simulink model "t_type_inverter"  (R2024b)
settings: Solver=FixedStepAuto  StartTime=0.0  StopTime=0.1  RelTol=1e-3
libraries: spsIGBTDiodeLib x12, spsVoltageMeasurementLib x3, spsDCVoltageSourceLib x2, spsGroundLib x1, spsThreePhaseSeriesRLCBranchLib x1, spsThreePhaseVIMeasurementLib x1, sps_lib x1
settings Model: Creator=Eng.Abd-Elrhman Saad  LastModifiedBy=Eng.Abd-Elrhman Saad

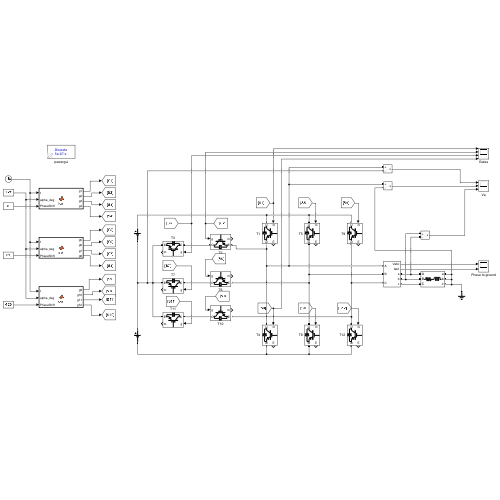
[thumbnail: Simulink's stored preview of the top-level diagram]
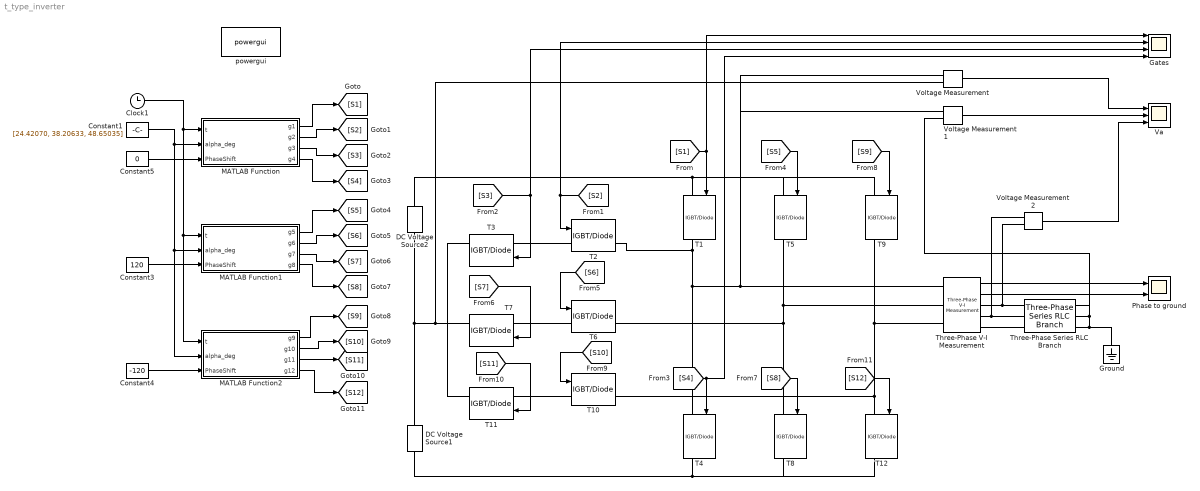
== system t_type_inverter ==
  Clock1 : Clock
  Constant1 : Constant  Value=[24.42070, 38.20633, 48.65035]
  Constant3 : Constant  Value=120
  Constant4 : Constant  Value=-120
  Constant5 : Constant  Value=0
  DC Voltage Source1 : spsDCVoltageSourceLib/DC Voltage Source  Amplitude=400  Measurements=None
  DC Voltage Source2 : spsDCVoltageSourceLib/DC Voltage Source  Amplitude=400  Measurements=None
  Gates : Scope  NumInputPorts=4
  Ground : spsGroundLib/Ground  LConnTagsString=a
  MATLAB Function : MATLAB Function  TreatAsAtomicUnit=on
  MATLAB Function1 : MATLAB Function  TreatAsAtomicUnit=on
  MATLAB Function2 : MATLAB Function  TreatAsAtomicUnit=on
  Phase to ground : Scope  NumInputPorts=2
  T{1..12} (12 alike) : spsIGBTDiodeLib/IGBT//Diode  Ron=1e-3  Rs=1e5  Cs=inf  Measurements=on
  Three-Phase Series RLC Branch : spsThreePhaseSeriesRLCBranchLib/Three-Phase Series RLC Branch  LConnTagsString=A|B|C  RConnTagsString=A|B|C  BranchType=RL  Resistance=7.07  Inductance=0.0225  Capacitance=1e-6  Measurements=None
  Three-Phase V-I Measurement : spsThreePhaseVIMeasurementLib/Three-Phase V-I Measurement  VoltageMeasurement=phase-to-ground  SetLabelV=off  LabelV=Vabc  Vpu=off  VpuLL=off  CurrentMeasurement=yes  SetLabelI=off  LabelI=Iabc  Ipu=off  Pbase=100e6  Vbase=500e3  OutputType=Complex  PhasorSimulation=off  PSBequivalent=0
  Va : Scope  NumInputPorts=3
  Voltage Measurement : spsVoltageMeasurementLib/Voltage Measurement  PhasorSimulation=off  OutputType=Complex  PSBequivalent=0
  Voltage Measurement1 : spsVoltageMeasurementLib/Voltage Measurement  PhasorSimulation=off  OutputType=Complex  PSBequivalent=0
  Voltage Measurement2 : spsVoltageMeasurementLib/Voltage Measurement  PhasorSimulation=off  OutputType=Complex  PSBequivalent=0
  powergui : sps_lib/powergui  Priority=1  SimulationMode=Discrete  SampleTime=5e-7  frequency=60  Iterations=50  frequencyindice=0  Pbase=100e6  ErrMax=1e-4  UnitsV=kV  UnitsW=MW  buscounter=0  FunctionMessages=off  echomessages=off  EnableUseOfTLC=off  CurrentSourceSwitches=off  DisableSnubberDevices=off  DisableRonSwitches=off  DisableVfSwitches=off  DisplayEquations=off  AutomaticDiscreteSolvers=off  SolverType=Tustin/Backward Euler (TBE)  Interpol=off  ExternalGateDelay=off  methode=off  Ts=100  x0status=blocks  SPID=on  SwTol=0  HookPort=off  NonlinearTolerance=1e-4  nMaxIteration=100  ContinueOnMaxIteration=off  RestoreLinks=warning  ResistiveCurrentMeasurement=off  Frange=[0:2:500]  Ylog=off  Xlog=on  ShowGrid=off  save=off  variable=ZData  structure=0  ZoomFFT=off  StartTime=0.0  cycles=1  DisplayStyle=1  fundamental=60  FreqAxis=off  MaxFrequency=1000  frequencyindicesteady=1  RmsSteady=1  display=off
  wires:
  MATLAB Function/1(g1) -> [S1]
  MATLAB Function/2(g2) -> [S2]
  MATLAB Function/3(g3) -> [S3]
  MATLAB Function/4(g4) -> [S4]
  MATLAB Function1/1(g5) -> [S5]
  MATLAB Function1/2(g6) -> [S6]
  MATLAB Function1/3(g7) -> [S7]
  MATLAB Function1/4(g8) -> [S8]
  MATLAB Function2/1(g9) -> [S9]
  MATLAB Function2/2(g10) -> [S10]
  MATLAB Function2/3(g11) -> [S11]
  MATLAB Function2/4(g12) -> [S12]
  [S1] -> Gates/1, T1/1
  [S2] -> Gates/2, T2/1
  [S3] -> Gates/3, T3/1
  [S4] -> Gates/4, T4/1
  [S5] -> T5/1
  [S6] -> T6/1
  [S7] -> T7/1
  [S8] -> T8/1
  [S9] -> T9/1
  [S10] -> T10/1
  [S11] -> T11/1
  [S12] -> T12/1
  Clock1/1 -> MATLAB Function2/1(t), MATLAB Function1/1(t), MATLAB Function/1(t)
  Constant1/1 -> MATLAB Function2/2(alpha_deg), MATLAB Function1/2(alpha_deg), MATLAB Function/2(alpha_deg)
  Constant5/1 -> MATLAB Function/3(PhaseShift)
  Constant4/1 -> MATLAB Function2/3(PhaseShift)
  Constant3/1 -> MATLAB Function1/3(PhaseShift)
  Voltage Measurement2/1 -> Va/3
  Voltage Measurement/1 -> Va/1
  Voltage Measurement1/1 -> Va/2
  Three-Phase V-I Measurement/1 -> Phase to ground/1
  Three-Phase V-I Measurement/2 -> Phase to ground/2
  connections:
  T1/LConn1 -- DC Voltage Source2/RConn1 -- T9/LConn1 -- T5/LConn1
  T1/RConn1 -- Voltage Measurement/LConn1 -- Voltage Measurement1/LConn1 -- Three-Phase V-I Measurement/LConn1 -- T4/LConn1 -- T2/RConn1
  T5/RConn1 -- Three-Phase V-I Measurement/LConn2 -- T8/LConn1 -- T6/RConn1
  T9/RConn1 -- Three-Phase V-I Measurement/LConn3 -- T10/RConn1 -- T12/LConn1
  T2/LConn1 -- T3/LConn1
  T6/LConn1 -- T7/LConn1
  T10/LConn1 -- T11/LConn1
  T12/RConn1 -- T8/RConn1 -- DC Voltage Source1/LConn1 -- T4/RConn1
  T11/RConn1 -- T3/RConn1 -- T7/RConn1 -- Voltage Measurement/LConn2 -- DC Voltage Source1/RConn1 -- DC Voltage Source2/LConn1
  Three-Phase V-I Measurement/RConn1 -- Three-Phase Series RLC Branch/LConn1 -- Voltage Measurement2/LConn2
  Three-Phase Series RLC Branch/LConn2 -- Voltage Measurement2/LConn1 -- Three-Phase V-I Measurement/RConn2
  Three-Phase V-I Measurement/RConn3 -- Three-Phase Series RLC Branch/LConn3
  Ground/LConn1 -- Three-Phase Series RLC Branch/RConn3 -- Three-Phase Series RLC Branch/RConn1 -- Voltage Measurement1/LConn2 -- Three-Phase Series RLC Branch/RConn2

== matlab function t_type_inverter/MATLAB Function ==
  data: t input; g1 output; alpha_deg input; g2 output; g3 output; g4 output; PhaseShift input
function [g1, g2, g3, g4] = fcn(t, alpha_deg, PhaseShift)
    % System Parameters
    Freq = 50; 
    w = 2*pi*Freq;
    
    % Calculate instantaneous phase angle (0 to 2pi)
    theta = mod(w*t + PhaseShift*(pi/180), 2*pi);
    
    % Convert switching angles to radians
    a = alpha_deg * (pi/180);
    a1 = a(1); a2 = a(2); a3 = a(3);
    
    % Initialize voltage state
    State = 0; 
    
    % --- PWM Logic (SHE Quarter-Wave Symmetry) ---
    if (theta < pi) 
        % Positive Half Cycle
        if (theta >= a1 && theta < a2) || ...
           (theta >= a3 && theta < (pi - a3)) || ...
           (theta >= (pi - a2) && theta < (pi - a1))
            State = 1;
        end
    else
        % Negative Half Cycle
        theta_rel = theta - pi;
        if (theta_rel >= a1 && theta_rel < a2) || ...
           (theta_rel >= a3 && theta_rel < (pi - a3)) || ...
           (theta_rel >= (pi - a2) && theta_rel < (pi - a1))
            State = -1;
        end
    end
    
    % --- Gate Signal Assignment (CORRECTED FOR T-TYPE) ---
    % T1: Top (Positive)
    % T4: Bottom (Negative)
    % T2 & T3: Middle (Neutral Path)
    
    g1 = 0; g2 = 0; g3 = 0; g4 = 0;
    
    switch State
        case 1      % Positive State (+Vdc/2)
            g1 = 1; 
            % In T-Type, T2/T3 must be OFF to prevent short to neutral
        case -1     % Negative State (-Vdc/2)
            g4 = 1; 
            % In T-Type, T2/T3 must be OFF
        otherwise   % Zero State (0V)
            % Current flows to/from neutral via T2 and T3
            g2 = 1; 
            g3 = 1;
    end
end

== matlab function t_type_inverter/MATLAB Function1 ==
  data: t input; g5 output; alpha_deg input; g6 output; g7 output; g8 output; PhaseShift input
function [g5, g6, g7, g8] = fcn(t, alpha_deg, PhaseShift)
    % System Parameters
    Freq = 50; 
    w = 2*pi*Freq;
    
    % Calculate instantaneous phase angle (0 to 2pi)
    theta = mod(w*t + PhaseShift*(pi/180), 2*pi);
    
    % Convert switching angles to radians
    a = alpha_deg * (pi/180);
    a1 = a(1); a2 = a(2); a3 = a(3);
    
    % Initialize voltage state
    State = 0; 
    
    % --- PWM Logic (SHE Quarter-Wave Symmetry) ---
    if (theta < pi) 
        % Positive Half Cycle
        if (theta >= a1 && theta < a2) || ...
           (theta >= a3 && theta < (pi - a3)) || ...
           (theta >= (pi - a2) && theta < (pi - a1))
            State = 1;
        end
    else
        % Negative Half Cycle
        theta_rel = theta - pi;
        if (theta_rel >= a1 && theta_rel < a2) || ...
           (theta_rel >= a3 && theta_rel < (pi - a3)) || ...
           (theta_rel >= (pi - a2) && theta_rel < (pi - a1))
            State = -1;
        end
    end
    
    % --- Gate Signal Assignment (CORRECTED FOR T-TYPE) ---
    % T1: Top (Positive)
    % T4: Bottom (Negative)
    % T2 & T3: Middle (Neutral Path)
    
    g5 = 0; g6 = 0; g7 = 0; g8 = 0;
    
    switch State
        case 1      % Positive State (+Vdc/2)
            g5 = 1; 
            % In T-Type, T2/T3 must be OFF to prevent short to neutral
        case -1     % Negative State (-Vdc/2)
            g8 = 1; 
            % In T-Type, T2/T3 must be OFF
        otherwise   % Zero State (0V)
            % Current flows to/from neutral via T2 and T3
            g6 = 1; 
            g7 = 1;
    end
end

== matlab function t_type_inverter/MATLAB Function2 ==
  data: g9 output; t input; g10 output; alpha_deg input; g11 output; g12 output; PhaseShift input
function [g9, g10, g11, g12] = fcn(t, alpha_deg, PhaseShift)
    % System Parameters
    Freq = 50; 
    w = 2*pi*Freq;
    
    % Calculate instantaneous phase angle (0 to 2pi)
    theta = mod(w*t + PhaseShift*(pi/180), 2*pi);
    
    % Convert switching angles to radians
    a = alpha_deg * (pi/180);
    a1 = a(1); a2 = a(2); a3 = a(3);
    
    % Initialize voltage state
    State = 0; 
    
    % --- PWM Logic (SHE Quarter-Wave Symmetry) ---
    if (theta < pi) 
        % Positive Half Cycle
        if (theta >= a1 && theta < a2) || ...
           (theta >= a3 && theta < (pi - a3)) || ...
           (theta >= (pi - a2) && theta < (pi - a1))
            State = 1;
        end
    else
        % Negative Half Cycle
        theta_rel = theta - pi;
        if (theta_rel >= a1 && theta_rel < a2) || ...
           (theta_rel >= a3 && theta_rel < (pi - a3)) || ...
           (theta_rel >= (pi - a2) && theta_rel < (pi - a1))
            State = -1;
        end
    end
    
    % --- Gate Signal Assignment (CORRECTED FOR T-TYPE) ---
    % T1: Top (Positive)
    % T4: Bottom (Negative)
    % T2 & T3: Middle (Neutral Path)
    
    g9 = 0; g10 = 0; g11 = 0; g12 = 0;
    
    switch State
        case 1      % Positive State (+Vdc/2)
            g9 = 1; 
            % In T-Type, T2/T3 must be OFF to prevent short to neutral
        case -1     % Negative State (-Vdc/2)
            g12 = 1; 
            % In T-Type, T2/T3 must be OFF
        otherwise   % Zero State (0V)
            % Current flows to/from neutral via T2 and T3
            g10 = 1; 
            g11 = 1;
    end
end
